simulink model "PHLOOP"  (Simulink 3.00)
settings: Solver=ode45  SolverMode=SingleTasking  StartTime=0.0  StopTime=10  MaxStep=0.010  RelTol=1e-3  AbsTol=1e-3
settings Model: TimeSaveName=t  SaveOutput=off

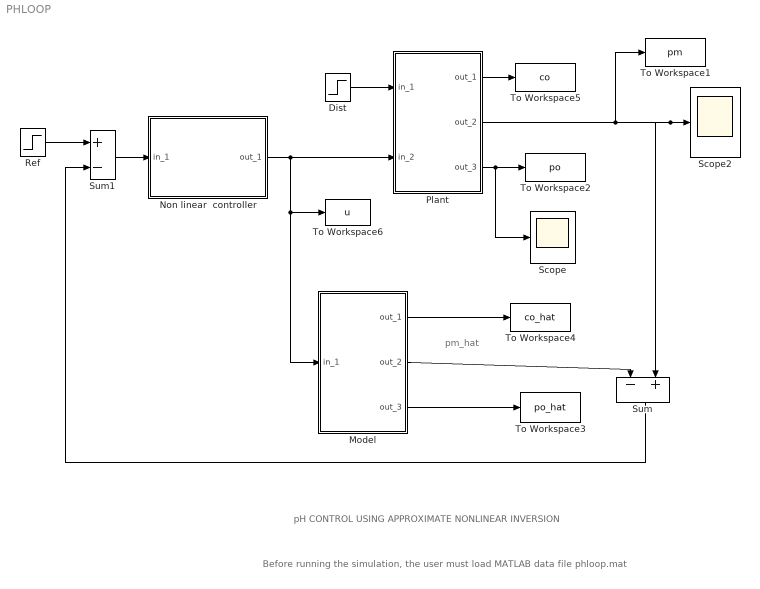
== system PHLOOP ==
  note: pm_hat
  note: pH CONTROL USING APPROXIMATE NONLINEAR INVERSION
  note: Before running the simulation, the user must load MATLAB data file phloop.mat
  Dist : Step  Time=5000  Before=0  After=0.000  SampleTime=0
  Model : Subsystem  mask(pH model){@1=V, @2=ci, @3=cu, @4=q, @5=alpha}
      mask prompts: @1 "Tank volume V:"; @2 "Inlet stream conc. ci:"; @3 "control acid stream conc. cu:"; @4 "inlet stream flow rate q:"; @5 "measurement  time constant alpha:"
      mask help: pH plant
      mask init:
      | V=@1;ci=@2;cu=@3;q=@4; alpha=@5;
      mask Display: disp('pH model')
  Non linear  controller : Subsystem  mask(Controller){@1=V, @2=ci, @3=cu, @4=q, @5=alpha, @6=beta}
      mask prompts: @1 "tank volume V:"; @2 "inlet stream conc. ci:"; @3 "control  stream conc. cu:"; @4 "inlet stream flow rate q:"; @5 "measurement tiem constant alpha:"; @6 "controller time constant beta:"
      mask help: Controller
      mask init:
      | V=@1;ci=@2;cu=@3;q=@4;alpha=@5;beta=@6;
      mask Display: disp('CONTROLLER')
  Plant : Subsystem  mask(pH plant){@1=V, @2=ci, @3=cu, @4=q, @5=alpha}
      mask prompts: @1 "Tank volume V:"; @2 "Inlet stream conc. ci:"; @3 "control acid stream conc. cu:"; @4 "inlet stream flow rate q:"; @5 "measurement  time constant alpha:"
      mask help: pH plant
      mask init:
      | V=@1;ci=@2;cu=@3;q=@4; alpha=@5;
      mask Display: disp('pH plant')
  Ref : Step  Time=2  Before=11  After=5  SampleTime=0
  Scope : Scope
      settings: TickLabels=on  TimeRange=10  YMin=0  YMax=14  SaveToWorkspace=off  SaveName=ScopeData  DataFormat=Matrix
  Scope2 : Scope
      settings: TickLabels=on  TimeRange=10  YMin=0  YMax=14  SaveToWorkspace=off  SaveName=ScopeData  DataFormat=Matrix
  Sum : Sum  Orientation=down  Inputs=-+  SaturateOnIntegerOverflow=on
  Sum1 : Sum  Inputs=+-  SaturateOnIntegerOverflow=on
  To Workspace1 : ToWorkspace  VariableName=pm  SampleTime=0  SaveFormat=Matrix
      settings: Buffer=10000
  To Workspace2 : ToWorkspace  VariableName=po  SampleTime=0  SaveFormat=Matrix
      settings: Buffer=10000
  To Workspace3 : ToWorkspace  VariableName=po_hat  SampleTime=0  SaveFormat=Matrix
      settings: Buffer=10000
  To Workspace4 : ToWorkspace  VariableName=co_hat  SampleTime=0  SaveFormat=Matrix
      settings: Buffer=10000
  To Workspace5 : ToWorkspace  VariableName=co  SampleTime=0  SaveFormat=Matrix
      settings: Buffer=10000
  To Workspace6 : ToWorkspace  VariableName=u  SampleTime=0  SaveFormat=Matrix
      settings: Buffer=10000
  wires:
  Model/2(out_2) -> Sum/1
  Model/3(out_3) -> To Workspace3/1
  Model/1(out_1) -> To Workspace4/1
  Ref/1 -> Sum1/1
  Plant/1(out_1) -> To Workspace5/1
  Sum1/1 -> Non linear  controller/1(in_1)
  Sum/1 -> Sum1/2
  Dist/1 -> Plant/1(in_1)
  Non linear  controller/1(out_1) -> Plant/2(in_2), Model/1(in_1), To Workspace6/1
  Plant/3(out_3) -> To Workspace2/1, Scope/1
  Plant/2(out_2) -> To Workspace1/1, Scope2/1, Sum/2

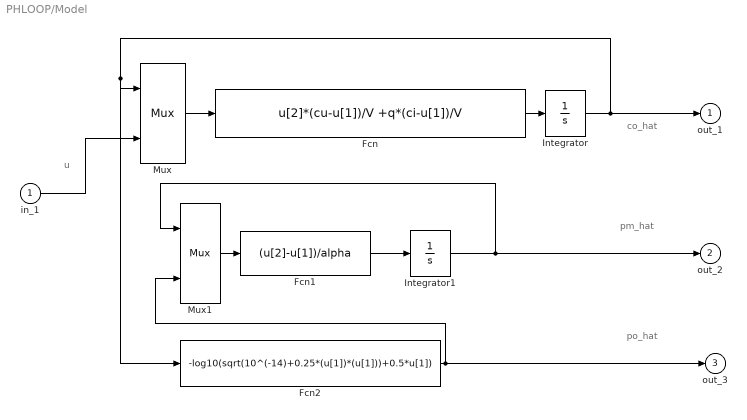
== system PHLOOP/Model ==
  note: pm_hat
  note: po_hat
  note: co_hat
  note: u
  in_1 : Inport  Port=1  PortWidth=-1  SampleTime=-1  DataType=auto
      settings: SignalType=auto
  Fcn : Fcn  Expr=u[2]*(cu-u[1])/V +q*(ci-u[1])/V
  Fcn1 : Fcn  Expr=(u[2]-u[1])/alpha
  Fcn2 : Fcn  Expr=-log10(sqrt(10^(-14)+0.25*(u[1])*(u[1]))+0.5*u[1])
  Integrator : Integrator  ExternalReset=none  InitialConditionSource=internal  InitialCondition=ci  LimitOutput=off  UpperSaturationLimit=inf  LowerSaturationLimit=-inf  ShowSaturationPort=off  ShowStatePort=off  AbsoluteTolerance=auto
  Integrator1 : Integrator  ExternalReset=none  InitialConditionSource=internal  InitialCondition=-log10(sqrt(10^(-14)+0.25*(ci)*(ci))+0.5*ci)  LimitOutput=off  UpperSaturationLimit=inf  LowerSaturationLimit=-inf  ShowSaturationPort=off  ShowStatePort=off  AbsoluteTolerance=auto
  Mux : Mux  Inputs=2
      settings: DisplayOption=none
  Mux1 : Mux  Inputs=2
      settings: DisplayOption=none
  out_1 : Outport  Port=1  InitialOutput=0
  out_2 : Outport  Port=2  InitialOutput=0
  out_3 : Outport  Port=3  InitialOutput=0
  wires:
  in_1/1 -> Mux/2
  Integrator/1 -> out_1/1, Mux/1, Fcn2/1
  Fcn2/1 -> out_3/1, Mux1/2
  Integrator1/1 -> out_2/1, Mux1/1
  Fcn1/1 -> Integrator1/1
  Mux1/1 -> Fcn1/1
  Fcn/1 -> Integrator/1
  Mux/1 -> Fcn/1

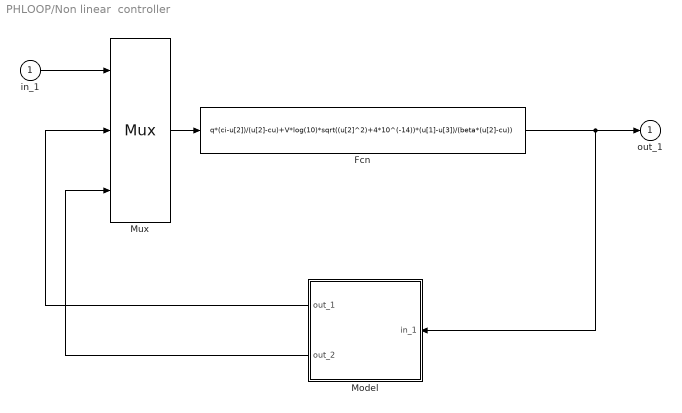
== system PHLOOP/Non linear  controller ==
  in_1 : Inport  Port=1  PortWidth=-1  SampleTime=-1  DataType=auto
      settings: SignalType=auto
  Fcn : Fcn  Expr=q*(ci-u[2])/(u[2]-cu)+V*log(10)*sqrt((u[2]^2)+4*10^(-14))*(u[1]-u[3])/(beta*(u[2]-cu))
  Model : Subsystem  Orientation=left
      mask Type: Model
      mask Display: disp('MODEL')
  Mux : Mux  Inputs=3
      settings: DisplayOption=none
  out_1 : Outport  Port=1  InitialOutput=0
  wires:
  Mux/1 -> Fcn/1
  in_1/1 -> Mux/1
  Model/1(out_1) -> Mux/2
  Model/2(out_2) -> Mux/3
  Fcn/1 -> out_1/1, Model/1(in_1)

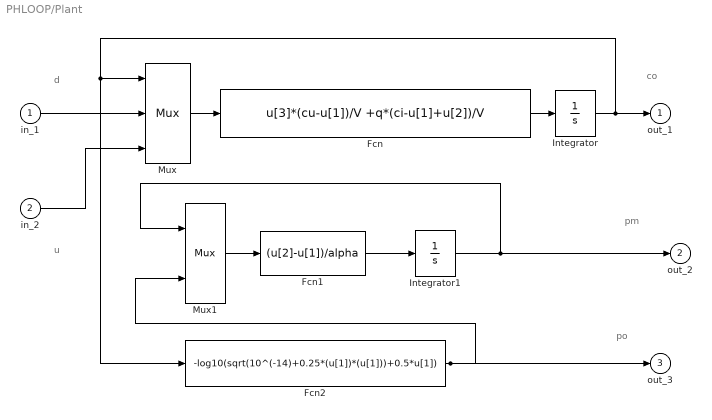
== system PHLOOP/Plant ==
  note: d
  note: u
  note: pm
  note: po
  note: co
  in_1 : Inport  Port=1  PortWidth=-1  SampleTime=-1  DataType=auto
      settings: SignalType=auto
  in_2 : Inport  Port=2  PortWidth=-1  SampleTime=-1  DataType=auto
      settings: SignalType=auto
  Fcn : Fcn  Expr=u[3]*(cu-u[1])/V +q*(ci-u[1]+u[2])/V
  Fcn1 : Fcn  Expr=(u[2]-u[1])/alpha
  Fcn2 : Fcn  Expr=-log10(sqrt(10^(-14)+0.25*(u[1])*(u[1]))+0.5*u[1])
  Integrator : Integrator  ExternalReset=none  InitialConditionSource=internal  InitialCondition=ci  LimitOutput=off  UpperSaturationLimit=inf  LowerSaturationLimit=-inf  ShowSaturationPort=off  ShowStatePort=off  AbsoluteTolerance=auto
  Integrator1 : Integrator  ExternalReset=none  InitialConditionSource=internal  InitialCondition=-log10(sqrt(10^(-14)+0.25*(ci)*(ci))+0.5*ci)  LimitOutput=off  UpperSaturationLimit=inf  LowerSaturationLimit=-inf  ShowSaturationPort=off  ShowStatePort=off  AbsoluteTolerance=auto
  Mux : Mux  Inputs=3
      settings: DisplayOption=none
  Mux1 : Mux  Inputs=2
      settings: DisplayOption=none
  out_1 : Outport  Port=1  InitialOutput=0
  out_2 : Outport  Port=2  InitialOutput=0
  out_3 : Outport  Port=3  InitialOutput=0
  wires:
  in_2/1 -> Mux/3
  in_1/1 -> Mux/2
  Mux/1 -> Fcn/1
  Fcn/1 -> Integrator/1
  Integrator/1 -> out_1/1, Mux/1, Fcn2/1
  Mux1/1 -> Fcn1/1
  Fcn1/1 -> Integrator1/1
  Integrator1/1 -> out_2/1, Mux1/1
  Fcn2/1 -> out_3/1, Mux1/2

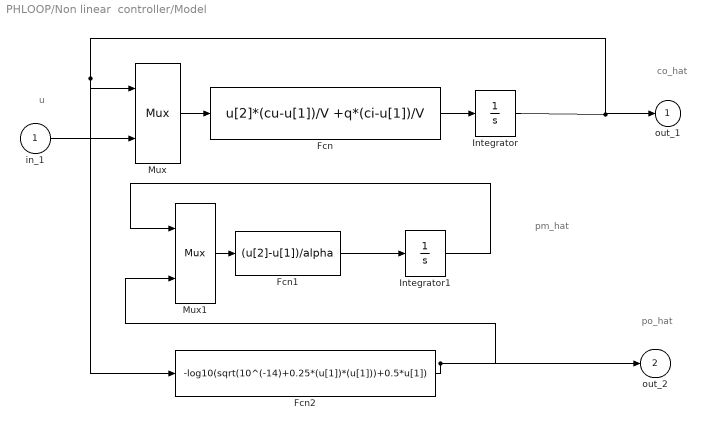
== system PHLOOP/Non linear  controller/Model ==
  note: po_hat
  note: co_hat
  note: u
  note: pm_hat
  in_1 : Inport  Port=1  PortWidth=-1  SampleTime=-1  DataType=auto
      settings: SignalType=auto
  Fcn : Fcn  Expr=u[2]*(cu-u[1])/V +q*(ci-u[1])/V
  Fcn1 : Fcn  Expr=(u[2]-u[1])/alpha
  Fcn2 : Fcn  Expr=-log10(sqrt(10^(-14)+0.25*(u[1])*(u[1]))+0.5*u[1])
  Integrator : Integrator  ExternalReset=none  InitialConditionSource=internal  InitialCondition=ci  LimitOutput=off  UpperSaturationLimit=inf  LowerSaturationLimit=-inf  ShowSaturationPort=off  ShowStatePort=off  AbsoluteTolerance=auto
  Integrator1 : Integrator  ExternalReset=none  InitialConditionSource=internal  InitialCondition=-log10(sqrt(10^(-14)+0.25*(ci)*(ci))+0.5*abs(ci))  LimitOutput=off  UpperSaturationLimit=inf  LowerSaturationLimit=-inf  ShowSaturationPort=off  ShowStatePort=off  AbsoluteTolerance=auto
  Mux : Mux  Inputs=2
      settings: DisplayOption=none
  Mux1 : Mux  Inputs=2
      settings: DisplayOption=none
  out_1 : Outport  Port=1  InitialOutput=0
  out_2 : Outport  Port=2  InitialOutput=0
  wires:
  in_1/1 -> Mux/2
  Integrator/1 -> out_1/1, Mux/1, Fcn2/1
  Fcn2/1 -> out_2/1, Mux1/2
  Integrator1/1 -> Mux1/1
  Fcn1/1 -> Integrator1/1
  Mux1/1 -> Fcn1/1
  Fcn/1 -> Integrator/1
  Mux/1 -> Fcn/1
